simulink model "simplifiedPWMandHalfBridge"  (R2014b)
settings: Solver=ode45  StartTime=0.0  StopTime=10.0  RelTol=1e-3
values from neighbouring files (symbols this model uses):
  Vcc = 24    [motorParams.m]

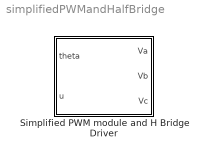
== system simplifiedPWMandHalfBridge ==
  Simplified PWM module and H Bridge Driver : Subsystem  mask{Vcc=Vcc}
      mask prompts: Vcc "Supply Voltage [V]:"
      mask help:
      | Input u = desired phase voltage
      |
      | Simulates the behavior of PWM generator and Half H Bridge Driver for the motor.
      |
      | The input voltage is taken in direcly as an input and is supplied voltage to the appropriate phase. The appropriate phase is determined by the rotor position and the 6-step BLDC commutation model.
      |
      | The high frequencies required to generate a true pwm signal that results in a smooth Vout slows down the simulation to a crawl, so it was approximated by this block.

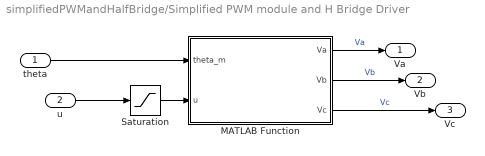
== system simplifiedPWMandHalfBridge/Simplified PWM module and H Bridge Driver ==
  theta : Inport
  u : Inport  Port=2
  MATLAB Function : MATLAB Function  TreatAsAtomicUnit=on  mask{poles=16}
      mask prompts: poles "Number of poles"
  Saturation : Saturate  UpperLimit=Vcc/2  LowerLimit=-Vcc/2
  Va : Outport
  Vb : Outport  Port=2
  Vc : Outport  Port=3
  wires:
  MATLAB Function/1(Va) -> Va/1  "Va"
  MATLAB Function/2(Vb) -> Vb/1  "Vb"
  MATLAB Function/3(Vc) -> Vc/1  "Vc"
  u/1 -> Saturation/1
  Saturation/1 -> MATLAB Function/2(u)
  theta/1 -> MATLAB Function/1(theta_m)

== matlab function simplifiedPWMandHalfBridge/Simplified PWM module and H Bridge Driver/MATLAB Function ==
function [Va, Vb, Vc] = halfBridge(theta_m, u)
    poles = 16;
    theta_e = (poles/2)*theta_m;
    theta_e = mod(theta_e, 2*pi);

    if theta_e <= pi/3
        Va = u/2;
        Vb = -u/2;
        Vc = 0;
    elseif theta_e <= 2*pi/3
        Va = u/2;
        Vb = 0;
        Vc = -u/2;
    elseif theta_e <= pi
        Va = 0;
        Vb = u/2;
        Vc = -u/2;
    elseif theta_e <= 4*pi/3
        Va = -u/2;
        Vb = u/2;
        Vc = 0;
    elseif theta_e <= 5*pi/3
        Va = -u/2;
        Vb = 0;
        Vc = u/2;
    else
        Va = 0;
        Vb = -u/2;
        Vc = u/2;
    end
end
